simulink model "sampleModel88"  (R2021b)
settings: Solver=VariableStepAuto  StartTime=0.0  StopTime=10.0  RelTol=1e-3
undefined symbols (not defined in the file or in its folder): DiscIntNeverNeededParam
libraries: simulink x4, slpidlib x1
settings Model: Creator=user  LastModifiedBy=user

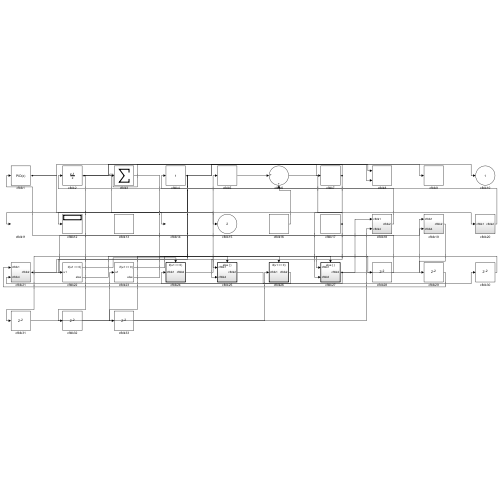
[thumbnail: Simulink's stored preview of the top-level diagram]
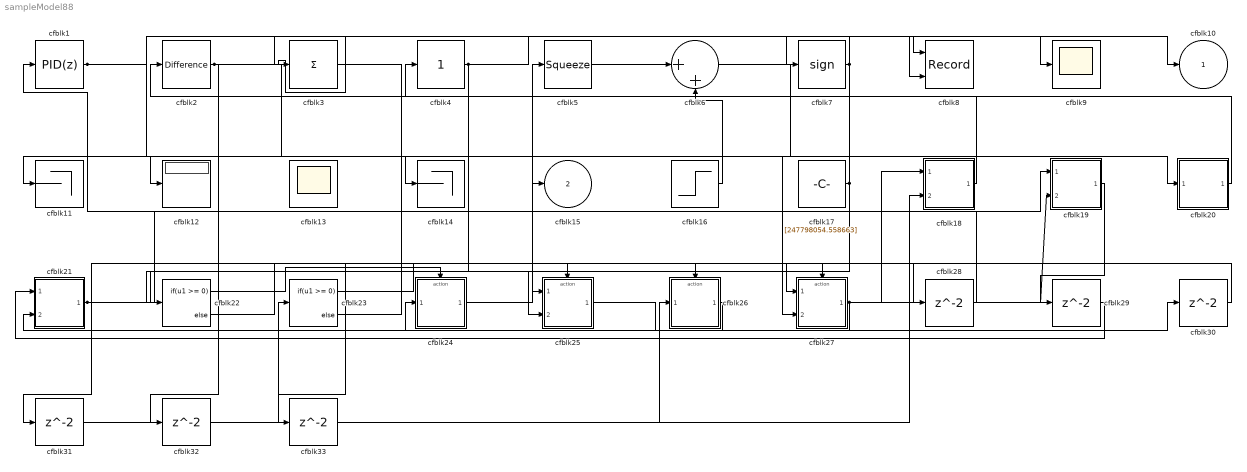
== system sampleModel88 ==
  cfblk1 : slpidlib/PID Controller  Controller=PID  Form=Parallel  TimeDomain=Discrete-time  UseExternalTs=off  SampleTime=1  IntegratorMethod=Forward Euler  FilterMethod=Forward Euler  ControllerParametersSource=internal  P=1  I=1  D=0  UseFilter=on  N=100  TunerSelectOption=Transfer Function Based (PID Tuner App)  InitialConditionSource=internal  InitialConditionForIntegrator=0  InitialConditionForFilter=0  DifferentiatorICPrevScaledInput=0  ExternalReset=none  TrackingMode=off  Kt=1  LimitOutput=off  SatLimitsSource=internal  UpperSaturationLimit=inf  LowerSaturationLimit=-inf  LinearizeAsGain=off  AntiWindupMode=none  Kb=1  POutMin=[]  POutMax=[]  IOutMin=[]  IOutMax=[]  DOutMin=[]  DOutMax=[]  NOutMin=[]  NOutMax=[]  SumOutMin=[]  SumOutMax=[]  SaturationOutMin=[]  SaturationOutMax=[]  PParamMin=[]  PParamMax=[]  IParamMin=[]  IParamMax=[]  DParamMin=[]  DParamMax=[]  NParamMin=[]  NParamMax=[]  KbParamMin=[]  KbParamMax=[]  KtParamMin=[]  KtParamMax=[]  KbOutMin=[]  KbOutMax=[]  KtOutMin=[]  KtOutMax=[]  IntegratorOutMin=[]  IntegratorOutMax=[]  FilterOutMin=[]  FilterOutMax=[]  SumI1OutMin=[]  SumI1OutMax=[]  SumI2OutMin=[]  SumI2OutMax=[]  SumI3OutMin=[]  SumI3OutMax=[]  SumI4OutMin=[]  SumI4OutMax=[]  SumDOutMin=[]  SumDOutMax=[]  DifferentiatorOutMin=[]  DifferentiatorOutMax=[]  FilterDiffOutCoefMin=[]  FilterDiffOutCoefMax=[]  ReciprocalOutMin=[]  ReciprocalOutMax=[]  SumDenOutMin=[]  SumDenOutMax=[]  SumNumOutMin=[]  SumNumOutMax=[]  DivideOutMin=[]  DivideOutMax=[]  UdiffTsProdOutMin=[]  UdiffTsProdOutMax=[]  NTsProdOutMin=[]  NTsProdOutMax=[]  UintegralTsProdOutMin=[]  UintegralTsProdOutMax=[]  UngainTsProdOutMin=[]  UngainTsProdOutMax=[]  IntegratorContinuousStateAttributes=''  IntegratorStateMustResolveToSignalObject=off  IntegratorRTWStateStorageClass=Auto  FilterContinuousStateAttributes=''  FilterStateMustResolveToSignalObject=off  FilterRTWStateStorageClass=Auto  ParallelPVariant=InternalParameters  IdealPVariant=Disabled  IVariant=InternalParameters  DVariant=InternalParameters  IntegratorVariant=Discrete  SatVariant=Disabled  AWVariant=Passthrough  PCopyVariant=Disabled  TRVariant=Disabled  FdbkBlocksVariant=Forward  IdealPFdbkVariant=Disabled  SatFdbkVariant=Disabled  DerivativeFilterVariant=ForwardEulerFilter  NVariant=InternalParameters  NCopyVariant=Disabled  FilterICVariant=InternalICsFilter  IntegratorICVariant=InternalICs  ExternalResetVariant=Disabled  TRSumVariant=Passthrough  SumFdbkVariant=Disabled  SumVariant=Sum_PID  TsampFilterVariant=InternalTs  TsampNgainVariant=Passthrough  TsampIntegralVariant=Passthrough  ExternalSaturationOutDataTypeStr=Inherit: Same as second input
  cfblk11 : Terminator
  cfblk12 : Display
  cfblk13 : Scope
      settings: Floating=on
  cfblk14 : Terminator
  cfblk16 : Step  Time=[42.000000]  Before=[-331244092.767330]  After=[91945921.940869]  SampleTime=0
  cfblk17 : Constant  Value=[247798054.558663]  SampleTime=1
  cfblk18 : Subsystem
  cfblk19 : Subsystem
  cfblk2 : simulink/Discrete/Difference  ICPrevInput=0.0  OutMin=[]  OutMax=[]  OutDataTypeStr=Inherit: Inherit via back propagation  OutDataType=fixdt(1, 16)  OutScaling=2^-10  DoSatur=off
  cfblk20 : Subsystem
  cfblk21 : Subsystem
  cfblk22 : If  IfExpression=u1 >= 0  SampleTime=1
  cfblk23 : If  IfExpression=u1 >= 0  SampleTime=1
  cfblk24 : Subsystem  TreatAsAtomicUnit=on
  cfblk25 : Subsystem  TreatAsAtomicUnit=on
  cfblk26 : Subsystem  TreatAsAtomicUnit=on
  cfblk27 : Subsystem  TreatAsAtomicUnit=on
  cfblk{28..33} (6 alike) : Delay  SampleTime=1
  cfblk3 : Sum  Inputs=+
  cfblk4 : simulink/Math Operations/Slider Gain  gain=1  low=0  high=2
  cfblk5 : Squeeze
  cfblk6 : Sum  Inputs=|++
  cfblk7 : Signum
  cfblk8 : Record  FileSettingsInternal="{\"entries\":[{\"content\":{\"excelSettings\":{\"content\":{},\"type\":\"Streamout.ExcelSettings\"}},\"type\":\"Streamout.FileSettingStorage\",\"uuid\":\"b038219a-e529-48f4-881b-4badf53b2b9a\"}],\"packageUris\":[\"http://schema.mathworks.com/mf0/streamout_blocks/R2020a\"],\"version\":\"1.0\"}"  Layout=[1 1]  SignalsInternal="{\"entries\":[{\"content\":{\"signals\":[{\"content\":{\"blockPath\":[\"sampleModel88/cfblk8\"],\"channel\":[],\"dimensions\":[1],\"domain\":\"sampleModel88/cfblk8\",\"lineColor\":\"#a2142f\",\"plots\":[1],\"port\":1,\"sid\":[\"\"],\"signalID\":3229,\"signalName\":\"cfblk2\"},\"type\":\"RecordBlkView.Signal\",\"uuid\":\"ab24b6fa-e36f-4130-b5ba-aebcd7f8bbcd\"},{\"content\":{\"blockPath\":[\"sampleModel88/cfblk8\"],\"channel\":[],\"dimensions\":[1],\"domain\":\"sampleModel88/cfblk8\",\"lineColor\":\"#139fff\",\"plots\":[1],\"port\":2,\"sid\":[\"\"],\"signalID\":3233,\"signalName\":\"cfblk4\"},\"type\":\"RecordBlkView.Signal\",\"uuid\":\"2c75b521-50e3-4ca5-921c-4dc232e13dc1\"}]},\"type\":\"RecordBlkView.InputSignals\",\"uuid\":\"449531fb-f29a-45db-ad19-62afd6d0b53e\"}],\"packageUris\":[\"http://schema.mathworks.com/mf0/streamout_blocks/R2020a\"],\"version\":\"1.0\"}"  VisualizationBindings="{\"xyplotplugin\":{\"info\":[{\"series\":[{\"bindingParametersList\":[{\"parameter\":\"X-Axis\",\"signalID\":3229,\"signalName\":\"cfblk2\"},{\"parameter\":\"Y-Axis\",\"signalID\":3233,\"signalName\":\"cfblk4\"}],\"seriesID\":13138}],\"subplotID\":1}]}}"  CompatibilityTag=XY
  cfblk9 : Scope
  cfblk10 : Outport
  cfblk15 : Outport  Port=2
  wires:
  cfblk5/1 -> cfblk6/1
  cfblk21/1(cfblk2) -> cfblk19/1(cfblk1), cfblk25/1(cfblk1)
  cfblk20/1(cfblk2) -> cfblk2/1
  cfblk24/1(cfblk2) -> cfblk5/1
  cfblk18/1(cfblk2) -> cfblk4/1
  cfblk2/1 -> cfblk15/1, cfblk8/1, cfblk10/1, cfblk32/1
  cfblk26/1(cfblk2) -> cfblk24/1(cfblk1)
  cfblk6/1 -> cfblk20/1(cfblk1)
  cfblk1/1 -> cfblk14/1, cfblk7/1
  cfblk17/1 -> cfblk11/1, cfblk25/2(cfblk4)
  cfblk4/1 -> cfblk22/1, cfblk9/1, cfblk12/1, cfblk8/2, cfblk31/1, cfblk33/1
  cfblk27/1(cfblk2) -> cfblk21/2(cfblk4), cfblk19/2(cfblk4), cfblk18/1(cfblk1)
  cfblk16/1 -> cfblk6/2
  cfblk7/1 -> cfblk3/1, cfblk27/2(cfblk3)
  cfblk22/1 -> cfblk24/Action
  cfblk22/2 -> cfblk25/Action
  cfblk23/1 -> cfblk26/Action
  cfblk23/2 -> cfblk27/Action
  cfblk3/1 -> cfblk28/1
  cfblk28/1 -> cfblk1/1
  cfblk19/1(cfblk2) -> cfblk29/1
  cfblk29/1 -> cfblk21/1(cfblk1)
  cfblk25/1(cfblk2) -> cfblk30/1
  cfblk30/1 -> cfblk27/1(cfblk1)
  cfblk31/1 -> cfblk26/1(cfblk1)
  cfblk32/1 -> cfblk23/1
  cfblk33/1 -> cfblk18/2(cfblk4)

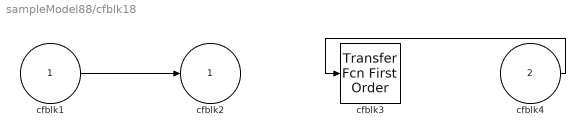
== system sampleModel88/cfblk18 ==
  cfblk1 : Inport
  cfblk4 : Inport  Port=2
  cfblk3 : simulink/Discrete/Transfer Fcn First Order  PoleZ=0.95  ICPrevOutput=0.0  DoSatur=off
  cfblk2 : Outport
  wires:
  cfblk4/1 -> cfblk3/1
  cfblk1/1 -> cfblk2/1

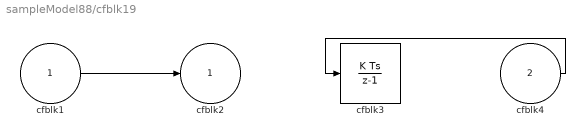
== system sampleModel88/cfblk19 ==
  cfblk1 : Inport
  cfblk4 : Inport  Port=2
  cfblk3 : DiscreteIntegrator  ICPrevOutput=DiscIntNeverNeededParam  ICPrevScaledInput=DiscIntNeverNeededParam
  cfblk2 : Outport
  wires:
  cfblk1/1 -> cfblk2/1
  cfblk4/1 -> cfblk3/1

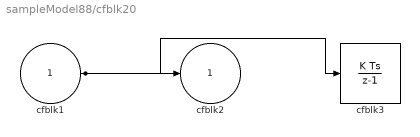
== system sampleModel88/cfblk20 ==
  cfblk1 : Inport
  cfblk3 : DiscreteIntegrator  ICPrevOutput=DiscIntNeverNeededParam  ICPrevScaledInput=DiscIntNeverNeededParam
  cfblk2 : Outport
  wires:
  cfblk1/1 -> cfblk2/1, cfblk3/1

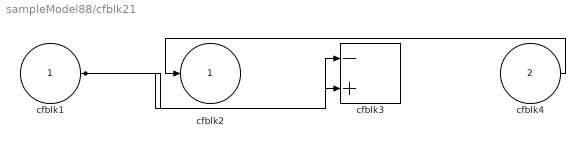
== system sampleModel88/cfblk21 ==
  cfblk1 : Inport
  cfblk4 : Inport  Port=2
  cfblk3 : Sum  Inputs=-+
  cfblk2 : Outport
  wires:
  cfblk4/1 -> cfblk2/1
  cfblk1/1 -> cfblk3/1, cfblk3/2

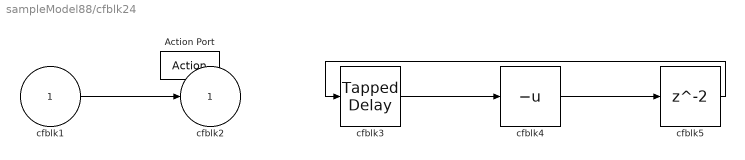
== system sampleModel88/cfblk24 ==
  cfblk1 : Inport
  Action Port : ActionPort  ActionPortLabel=if(u1 >= 0)
  cfblk3 : simulink/Discrete/Tapped Delay  vinit=0.0  samptime=-1  NumDelays=1  DelayOrder=Oldest  includeCurrent=off
  cfblk4 : UnaryMinus
  cfblk5 : Delay
  cfblk2 : Outport
  wires:
  cfblk1/1 -> cfblk2/1
  cfblk3/1 -> cfblk4/1
  cfblk4/1 -> cfblk5/1
  cfblk5/1 -> cfblk3/1

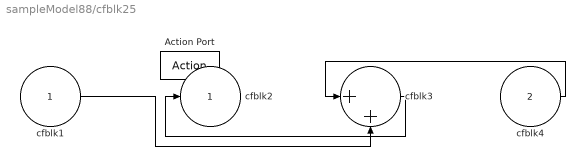
== system sampleModel88/cfblk25 ==
  cfblk1 : Inport
  cfblk4 : Inport  Port=2
  Action Port : ActionPort  ActionPortLabel=else
  cfblk3 : Sum  Inputs=|++
  cfblk2 : Outport
  wires:
  cfblk4/1 -> cfblk3/1
  cfblk3/1 -> cfblk2/1
  cfblk1/1 -> cfblk3/2

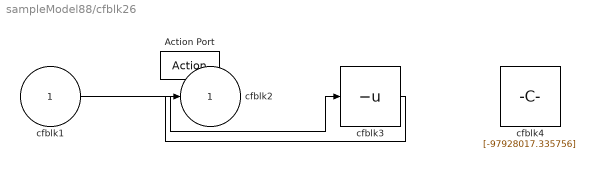
== system sampleModel88/cfblk26 ==
  cfblk1 : Inport
  Action Port : ActionPort  ActionPortLabel=if(u1 >= 0)
  cfblk3 : UnaryMinus
  cfblk4 : Constant  Value=[-97928017.335756]  SampleTime=1
  cfblk2 : Outport
  wires:
  cfblk1/1 -> cfblk3/1
  cfblk3/1 -> cfblk2/1

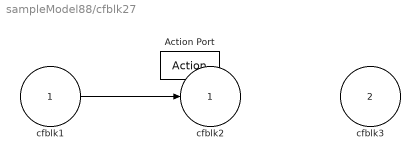
== system sampleModel88/cfblk27 ==
  cfblk1 : Inport
  cfblk3 : Inport  Port=2
  Action Port : ActionPort  ActionPortLabel=else
  cfblk2 : Outport
  wires:
  cfblk1/1 -> cfblk2/1
